simulink model "SYDE_351_Project_Suspension"  (R2023a)
settings: Solver=VariableStepAuto  StartTime=0.0  StopTime=15  RelTol=1e-3  AbsTol=1e-3
values from neighbouring files (symbols this model uses):
  C = C_array(j)    [iterations.m]
  LC = 20    [SYDE_351_Project_Parameters.m]
  M = 20    [SYDE_351_Project_Parameters.m]
libraries: fl_lib x7, nesl_utility x4, simulink x1
settings Model: Creator=danielkang  LastModifiedBy=rayan
settings SolverCC: AutoScaleAbsTol=off  AlgebraicLoopSolver=TrustRegion  MaxZcPerStep=1
settings OptimizationCC: ReuseModelBlockBuffer=off
settings DebuggingCC: UnconnectedInputMsg=warning  UnconnectedOutputMsg=warning  UnconnectedLineMsg=warning  SymbolicDimsDataTypeCodeGenerationDiagnostic=none
settings ModelReferenceCC: EnableRefExpFcnMdlSchedulingChecks=on
settings SFSimCC: CustomCodeUndefinedFunction=UseInterfaceOnly
settings RTWCC: DLArmComputeVersion=19.05
settings SimscapeCC: SimscapeLogType=all  SimscapeLogSimulationStatistics=on  SimscapeLogDataHistory=10000

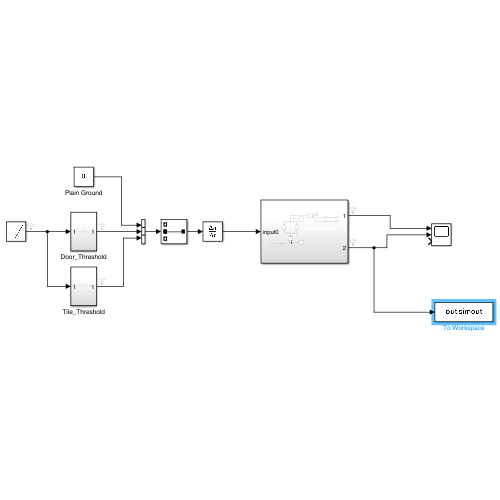
[thumbnail: Simulink's stored preview of the top-level diagram]
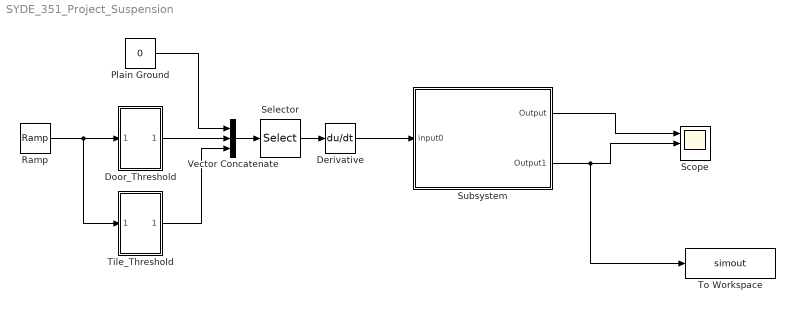
== system SYDE_351_Project_Suspension ==
  Derivative : Derivative
  Door_Threshold : Subsystem
  Plain Ground : Constant  Value=0
  Ramp : simulink/Sources/Ramp  slope=1/3  start=0  InitialOutput=0
  Scope : Scope  NumInputPorts=3
  Selector : Selector  InputPortWidth=3  IndexOptions=Index vector (dialog)  Indices=[2]  OutputSizes=1
  Subsystem : Subsystem
  Tile_Threshold : Subsystem
  To Workspace : ToWorkspace  VariableName=simout  SaveFormat=Timeseries  SampleTime=-1
  Vector Concatenate : Concatenate  NumInputs=3
  wires:
  Ramp/1 -> Tile_Threshold/1(In1), Door_Threshold/1(In1)
  Selector/1 -> Derivative/1
  Door_Threshold/1(Output) -> Vector Concatenate/2
  Plain Ground/1 -> Vector Concatenate/1
  Tile_Threshold/1(Out1) -> Vector Concatenate/3
  Vector Concatenate/1 -> Selector/1
  Derivative/1 -> Subsystem/1(input0)
  Subsystem/1(Output) -> Scope/1
  Subsystem/2(Output1) -> To Workspace/1, Scope/2

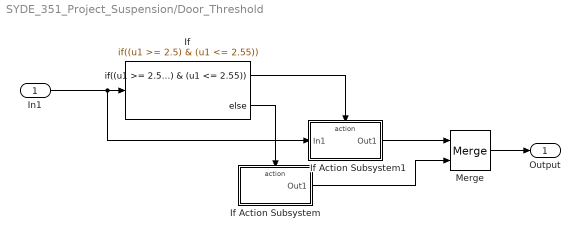
== system SYDE_351_Project_Suspension/Door_Threshold ==
  In1 : Inport
  If : If  IfExpression=(u1 >= 2.5) & (u1 <= 2.55)
  If Action Subsystem : Subsystem  TreatAsAtomicUnit=on
  If Action Subsystem1 : Subsystem  TreatAsAtomicUnit=on
  Merge : Merge
  Output : Outport
  wires:
  In1/1 -> If Action Subsystem1/1(In1), If/1
  If/1 -> If Action Subsystem1/Action
  If/2 -> If Action Subsystem/Action
  If Action Subsystem1/1(Out1) -> Merge/1
  If Action Subsystem/1(Out1) -> Merge/2
  Merge/1 -> Output/1

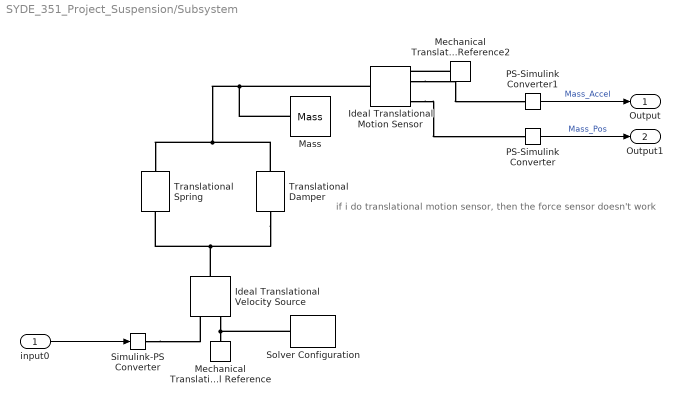
== system SYDE_351_Project_Suspension/Subsystem ==
  note: if i do translational motion sensor, then the force sensor doesn't work
  input0 : Inport
  Ideal Translational Motion Sensor : fl_lib/Mechanical/Mechanical Sensors/Ideal Translational Motion Sensor  reference=foundation.enum.MeasurementReference.difference  acceleration_port=true  velocity_port=true  position_port=true  offset=0 m
      settings: InternalSimscapePortConfiguration="{\"Bottom\":[],\"Left\":[{\"id\":\"R\",\"label\":\"R\",\"type\":\"foundation.mechanical.translational.translational\"}],\"Right\":[{\"id\":\"C\",\"label\":\"C\",\"type\":\"foundation.mechanical.translational.translational\"},{\"id\":\"A\",\"label\":\"A\",\"type\":\"output\"},{\"id\":\"V\",\"label\":\"V\",\"type\":\"output\"},{\"id\":\"P\",\"label\":\"P\",\"type\":\"output\"}],\"Top\":[]}"
  Ideal Translational Velocity Source : fl_lib/Mechanical/Mechanical Sources/Ideal Translational Velocity Source
  Mass : fl_lib/Mechanical/Translational Elements/Mass  mass=M+LC kg  num_ports=foundation.enum.numPorts2.one  v_specify=off  v_priority=High  v=0 m/s  v_nominal_specify=off  v_nominal_unit=m/s  v_nominal_value=1  f_specify=off  f_priority=None  f=0 N  f_nominal_specify=off  f_nominal_unit=N  f_nominal_value=1
  Mechanical Translational Reference : fl_lib/Mechanical/Translational Elements/Mechanical Translational Reference
  Mechanical Translational Reference2 : fl_lib/Mechanical/Translational Elements/Mechanical Translational Reference
  PS-Simulink Converter : nesl_utility/PS-Simulink Converter  PhysicalDomain=network_engine_domain  SubClassName=ps_output  LeftPortType=input  RightPortType=output  PseudoPeriodic=off  Frequencies=[]  VectorFormat=inherit  Unit=inherit  AffineConversion=off
  PS-Simulink Converter1 : nesl_utility/PS-Simulink Converter  PhysicalDomain=network_engine_domain  SubClassName=ps_output  LeftPortType=input  RightPortType=output  PseudoPeriodic=off  Frequencies=[]  VectorFormat=inherit  Unit=inherit  AffineConversion=off
  Simulink-PS Converter : nesl_utility/Simulink-PS Converter  PhysicalDomain=network_engine_domain  SubClassName=ps_input  LeftPortType=input  RightPortType=output  PseudoPeriodic=off  Frequencies=[]  NoiseDistribution=none  NoiseParameters=[]  Unit=m/s  AffineConversion=off  FilteringAndDerivatives=provide  SimscapeFilterOrder=1  InputFilterTimeConstant=0.001  UdotUserProvided=0
  Solver Configuration : nesl_utility/Solver Configuration  PhysicalDomain=network_engine_domain  SubClassName=solver  LeftPortType=input  RightPortType=generic  Tones=[]  Harmonics=[]  SimulateNoise=off  Profile=off  UseLocalSampling=off  EnableSwitchedLinearOptims=on  FrequencyDomain=off  UseCCode=off  RelTol=0.001  AbsTol=1e-06  MinStep=1e-09  ToWorkspace=off  RevertToSquareIcSolve=off  NumHomotopyIterations=100  PhasorMode=off  PhasorModeNumHarmonics=1  ConsistencySolver=NEWTON_XTOL_AFTER_FTOL  IndexReductionMethod=DerivativeReplacement  DoDC=off  ResidualTolerance=1e-09  ConsistencyTolSource=GLOBAL  ConsistencyAbsTol=0.001  ConsistencyRelTol=0.001  ConsistencyTolFactor=0.001  UseLocalSolver=off  LocalSolverChoice=NE_BACKWARD_EULER_ADVANCER  ResolveIndetEquations=on  FunctionEvalNumThread=1  LocalSolverSampleTime=0.001  DoFixedCost=off  MaxNonlinIter=3  MaxModeIter=2  ComputeImpulses=off  ImpulseIterations=2  LinearAlgebra=auto  LinearAlgebraNumThread=0  EquationFormulation=NE_TIME_EF  DelaysMemoryBudget=1024  AutomaticFiltering=on  FilteringTimeConstant=0.001  PartitionStorageMethod=AS_NEEDED  PartitionMemoryBudget=1024  PartitionMethod=ROBUST
  Translational Damper : fl_lib/Mechanical/Translational Elements/Translational Damper  D=C N*s/m  v_specify=off  v_priority=None  v=0 m/s  v_nominal_specify=off  v_nominal_unit=m/s  v_nominal_value=1  f_specify=off  f_priority=None  f=0 N  f_nominal_specify=off  f_nominal_unit=N  f_nominal_value=1
  Translational Spring : fl_lib/Mechanical/Translational Elements/Translational Spring  spr_rate=K N/m  v_specify=off  v_priority=None  v=0 m/s  v_nominal_specify=off  v_nominal_unit=m/s  v_nominal_value=1  f_specify=off  f_priority=None  f=0 N  f_nominal_specify=off  f_nominal_unit=N  f_nominal_value=1  x_specify=off  x_priority=High  x=0 m  x_nominal_specify=off  x_nominal_unit=m  x_nominal_value=1
  Output : Outport
  Output1 : Outport  Port=2
  wires:
  input0/1 -> Simulink-PS Converter/1
  PS-Simulink Converter1/1 -> Output/1  "Mass_Accel"
  PS-Simulink Converter/1 -> Output1/1  "Mass_Pos"
  connections:
  Simulink-PS Converter/RConn1 -- Ideal Translational Velocity Source/RConn1
  Mass/LConn1 -- Translational Damper/LConn1 -- Translational Spring/LConn1 -- Ideal Translational Motion Sensor/LConn1
  Ideal Translational Velocity Source/RConn2 -- Mechanical Translational Reference/LConn1 -- Solver Configuration/RConn1
  Translational Damper/RConn1 -- Ideal Translational Velocity Source/LConn1 -- Translational Spring/RConn1
  Ideal Translational Motion Sensor/RConn2 -- PS-Simulink Converter1/LConn1
  Ideal Translational Motion Sensor/RConn4 -- PS-Simulink Converter/LConn1
  Mechanical Translational Reference2/LConn1 -- Ideal Translational Motion Sensor/RConn1

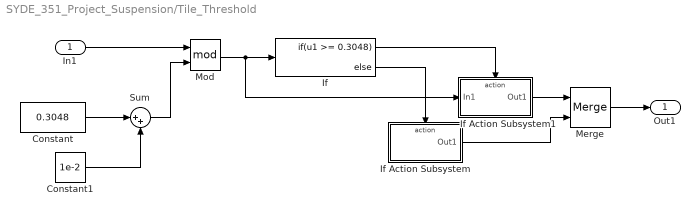
== system SYDE_351_Project_Suspension/Tile_Threshold ==
  In1 : Inport
  Constant : Constant  Value=0.3048
  Constant1 : Constant  Value=1e-2
  If : If  IfExpression=u1 >= 0.3048
  If Action Subsystem : Subsystem  TreatAsAtomicUnit=on
  If Action Subsystem1 : Subsystem  TreatAsAtomicUnit=on
  Merge : Merge
  Mod : Math  Operator=mod
  Sum : Sum  Inputs=|++
  Out1 : Outport
  wires:
  If/1 -> If Action Subsystem1/Action
  If/2 -> If Action Subsystem/Action
  In1/1 -> Mod/1
  Mod/1 -> If Action Subsystem1/1(In1), If/1
  Constant/1 -> Sum/1
  Sum/1 -> Mod/2
  Constant1/1 -> Sum/2
  If Action Subsystem1/1(Out1) -> Merge/1
  If Action Subsystem/1(Out1) -> Merge/2
  Merge/1 -> Out1/1

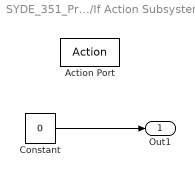
== system SYDE_351_Project_Suspension/Door_Threshold/If Action Subsystem ==
  Action Port : ActionPort  ActionPortLabel=else
  Constant : Constant  Value=0
  Out1 : Outport
  wires:
  Constant/1 -> Out1/1

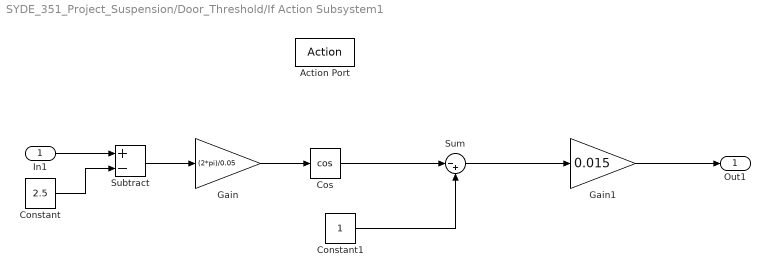
== system SYDE_351_Project_Suspension/Door_Threshold/If Action Subsystem1 ==
  In1 : Inport
  Action Port : ActionPort  ActionPortLabel=if((u1 >= 2.5) & (u1 <= 2.55))
  Constant : Constant  Value=2.5
  Constant1 : Constant
  Cos : Trigonometry  Operator=cos
  Gain : Gain  Gain=(2*pi)/0.05
  Gain1 : Gain  Gain=0.015
  Subtract : Sum  Inputs=+-
  Sum : Sum  Inputs=|-+
  Out1 : Outport
  wires:
  Sum/1 -> Gain1/1
  Gain1/1 -> Out1/1
  Cos/1 -> Sum/1
  Constant1/1 -> Sum/2
  Gain/1 -> Cos/1
  Constant/1 -> Subtract/2
  Subtract/1 -> Gain/1
  In1/1 -> Subtract/1

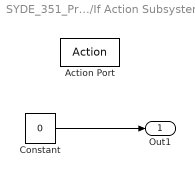
== system SYDE_351_Project_Suspension/Tile_Threshold/If Action Subsystem ==
  Action Port : ActionPort  ActionPortLabel=else
  Constant : Constant  Value=0
  Out1 : Outport
  wires:
  Constant/1 -> Out1/1

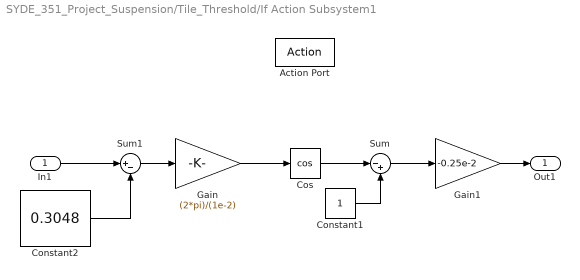
== system SYDE_351_Project_Suspension/Tile_Threshold/If Action Subsystem1 ==
  In1 : Inport
  Action Port : ActionPort  ActionPortLabel=if(u1 >= 0.3048)
  Constant1 : Constant
  Constant2 : Constant  Value=0.3048
  Cos : Trigonometry  Operator=cos
  Gain : Gain  Gain=(2*pi)/(1e-2)
  Gain1 : Gain  Gain=-0.25e-2
  Sum : Sum  Inputs=|-+
  Sum1 : Sum  Inputs=|+-
  Out1 : Outport
  wires:
  Sum/1 -> Gain1/1
  Gain1/1 -> Out1/1
  Cos/1 -> Sum/1
  Constant1/1 -> Sum/2
  Gain/1 -> Cos/1
  Sum1/1 -> Gain/1
  In1/1 -> Sum1/1
  Constant2/1 -> Sum1/2
